simulink model "six_dof_BACK_STEPPING"  (R2021b)
settings: Solver=ode4  StartTime=0.0  StopTime=10.0  FixedStep=0.01  RelTol=1e-3
libraries: robotmaniplib x5, simulink x2
settings Model: Creator=marco  LastModifiedBy=marco

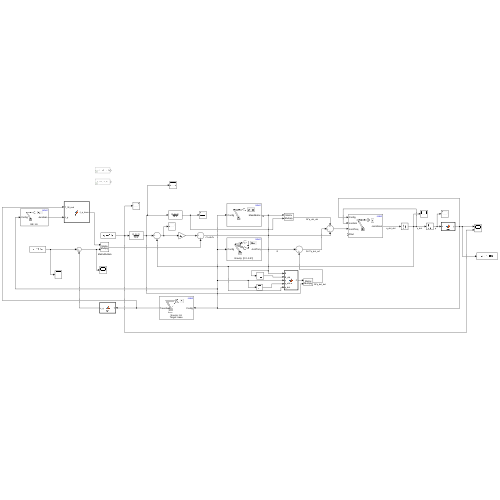
[thumbnail: Simulink's stored preview of the top-level diagram]
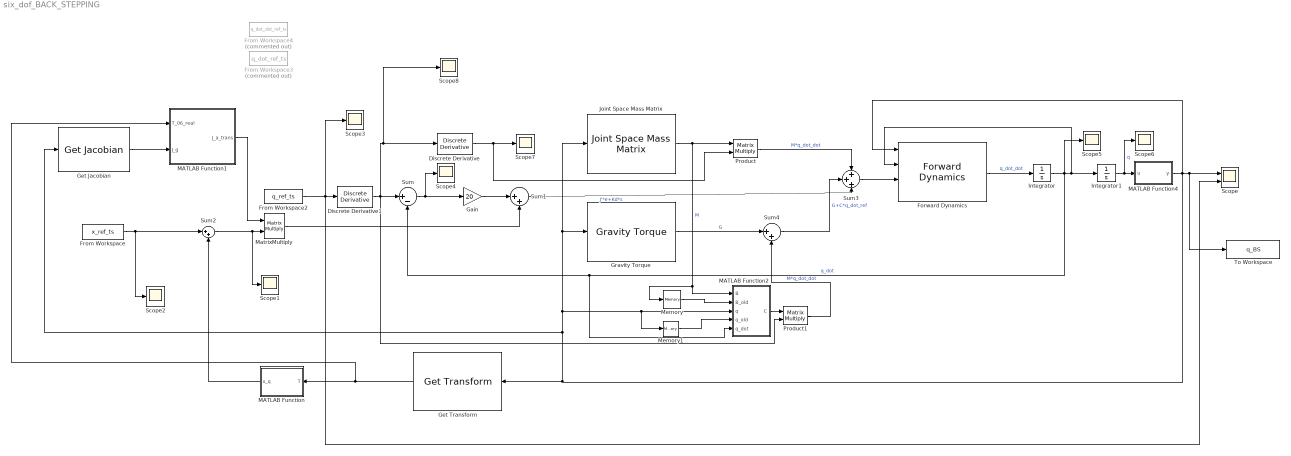
== system six_dof_BACK_STEPPING ==
  Discrete Derivative : simulink/Discrete/Discrete Derivative  gainval=1.0  ICPrevScaledInput=0.0  OutMin=[]  OutMax=[]  OutDataType=fixdt(1, 16)  OutScaling=2^-10  DoSatur=off
  Discrete Derivative1 : simulink/Discrete/Discrete Derivative  gainval=1.0  ICPrevScaledInput=0.0  OutMin=[]  OutMax=[]  OutDataType=fixdt(1, 16)  OutScaling=2^-10  DoSatur=off
  Forward Dynamics : robotmaniplib/Forward Dynamics  RigidBodyTree=robot  SimulateUsing=Interpreted execution
  From Workspace : FromWorkspace  VariableName=x_ref_ts
  From Workspace2 : FromWorkspace  VariableName=q_ref_ts
  From Workspace3 : FromWorkspace  Commented=on  VariableName=q_dot_ref_ts
  From Workspace4 : FromWorkspace  Commented=on  VariableName=q_dot_dot_ref_ts
  Gain : Gain  Gain=20
  Get Jacobian : robotmaniplib/Get Jacobian  RigidBodyTree=robot  EndEffector=L6  SimulateUsing=Interpreted execution
      settings: SourceProductBaseCode=RO
  Get Transform : robotmaniplib/Get Transform  RigidBodyTree=robot  SourceBody=L6  TargetBody=base  SimulateUsing=Interpreted execution
  Gravity Torque : robotmaniplib/Gravity Torque  RigidBodyTree=robot  SimulateUsing=Interpreted execution
  Integrator : Integrator  InitialCondition=[0; 0; 0; 0; 0; 0]  LimitOutput=on  UpperSaturationLimit=[pi/2; pi/2; pi/2; pi/2; pi/2; pi/2]  LowerSaturationLimit=-[pi/2; pi/2; pi/2; pi/2; pi/2; pi/2]
  Integrator1 : Integrator  InitialCondition=[0; 0; 0; 0; pi/2; 0]  LimitOutput=on  UpperSaturationLimit=[pi; pi/4; 5*pi/4; pi; 5*pi/4; pi]  LowerSaturationLimit=-[pi; 5*pi/4; pi/4; pi; 5*pi/4; pi]
  Joint Space Mass Matrix : robotmaniplib/Joint Space Mass Matrix  RigidBodyTree=robot  SimulateUsing=Interpreted execution
  MATLAB Function : MATLAB Function  TreatAsAtomicUnit=on
  MATLAB Function1 : MATLAB Function  TreatAsAtomicUnit=on
  MATLAB Function2 : MATLAB Function  TreatAsAtomicUnit=on
  MATLAB Function4 : MATLAB Function  TreatAsAtomicUnit=on
  MatrixMultiply : Product  Multiplication=Matrix(*)
  Memory : Memory
  Memory1 : Memory
  Product : Product  Multiplication=Matrix(*)
  Product1 : Product  Multiplication=Matrix(*)
  Scope : Scope  NumInputPorts=2
  Scope{1..8} (8 alike) : Scope
  Sum : Sum  Inputs=|+-
  Sum1 : Sum  Inputs=|++
  Sum2 : Sum  Inputs=|++
  Sum3 : Sum  Inputs=+++
  Sum4 : Sum  Inputs=|++
  To Workspace : ToWorkspace  VariableName=q_BS  SaveFormat=Timeseries  SampleTime=-1
  wires:
  Discrete Derivative1/1 -> Sum/1, Product1/2, Scope8/1, Discrete Derivative/1
  Integrator1/1 -> Scope6/1, MATLAB Function4/1(u)  "q"
  From Workspace2/1 -> Scope3/1, Discrete Derivative1/1, Scope/2
  Sum3/1 -> Forward Dynamics/3
  Gravity Torque/1 -> Sum4/1  "G"
  Sum4/1 -> Sum3/2  "G+C*q_dot_ref"
  MATLAB Function4/1(y) -> Joint Space Mass Matrix/1, Gravity Torque/1, MATLAB Function2/3(q), Memory1/1, Get Jacobian/1, Get Transform/1, To Workspace/1, Scope/1, Forward Dynamics/1
  Forward Dynamics/1 -> Integrator/1  "q_dot_dot"
  Integrator/1 -> Scope5/1, Forward Dynamics/2, Integrator1/1, MATLAB Function2/5(q_dot), Sum/2  "q_dot"
  Sum/1 -> Scope4/1, Gain/1
  Product/1 -> Sum3/1  "M*q_dot_dot"
  Discrete Derivative/1 -> Product/2, Scope7/1
  Gain/1 -> Sum1/1
  Sum1/1 -> Sum3/3  "J'*e+Kd*s"
  Get Transform/1 -> MATLAB Function1/1(T_06_real), MATLAB Function/1(T)
  MATLAB Function/1(x_q) -> Sum2/2
  From Workspace/1 -> Sum2/1, Scope2/1
  Joint Space Mass Matrix/1 -> Memory/1, MATLAB Function2/1(B), Product/1  "M"
  MATLAB Function1/1(J_a_trans) -> MatrixMultiply/1
  Sum2/1 -> Scope1/1, MatrixMultiply/2
  MatrixMultiply/1 -> Sum1/2
  Get Jacobian/1 -> MATLAB Function1/2(J_g)
  MATLAB Function2/1(C) -> Product1/1
  Product1/1 -> Sum4/2  "M*q_dot_dot"
  Memory/1 -> MATLAB Function2/2(B_old)
  Memory1/1 -> MATLAB Function2/4(q_old)

== matlab function six_dof_BACK_STEPPING/MATLAB Function2 ==
  settings: updateMethod=DISCRETE
  data: B input; B_old input; C output; q input; q_old input; q_dot input
function C = fcn(B, B_old, q, q_old, q_dot)

% persistent B_old q_old 
 C = zeros(6,6);
% if isempty(q_old)
%     step = deg2rad(1);
%     q_old = [-step; -step; -step; -step; pi/2-step; -step];
%     B_old = B;
     c = zeros(6,6,6);
% end

for i=1:6
    for j=1:6
        for k=1:6
            c(i,j,k) = 1/2*((B(i,j)-B_old(i,j))/(q(k)-q_old(k))+(B(i,k)-B_old(i,k))/(q(j)-q_old(j))-(B(j,k)-B_old(j,k))/(q(i)-q_old(i)));
            C(i,j)=C(i,j)+c(i,j,k)*q_dot(k);
        end
    end
end

% B_old = B;
% q_old = q;

== matlab function six_dof_BACK_STEPPING/MATLAB Function ==
  data: T input; x_q output
function x_q = fcn(T)
angle = tform2eul(T);
x_q = [T(1:3,4); angle'];

== matlab function six_dof_BACK_STEPPING/MATLAB Function1 ==
  data: T_06_real input; J_a_trans output; J_g input
function J_a_trans = fcn(T_06_real, J_g)

angl=tform2eul(T_06_real);

% T_w_phi = [cos(angl(1))*cos(angl(2))   -sin(angl(1))   0
%            sin(angl(1))*cos(angl(2))   cos(angl(1))    0
%            -sin(angl(2))               0               1];

T_w_phi = [0 -sin(angl(1)) cos(angl(1))*cos(angl(2))   
           0  cos(angl(1)) sin(angl(1))*cos(angl(2))
           1  0            -sin(angl(2))            ];

T_a=blkdiag(eye(3),T_w_phi);

J_a=T_a\J_g;

J_a_trans = J_a';

end

== matlab function six_dof_BACK_STEPPING/MATLAB Function4 ==
  data: u input; y output
function y = fcn(u)

y = wrapToPi(u);
